simulink subsystem "Lib_QuinIDRxDDC"  (R2023b)
settings: Solver=VariableStepAuto  StartTime=0.0  StopTime=10.0  RelTol=1e-3
values from neighbouring files (symbols this model uses):
  FILT = getFilters(SRC)    [Initialize.m]
undefined symbols (not defined in the file or in its folder): ReaderReceive
libraries: dsphdlfiltering2 x42
settings Model: Creator=NaXin  LastModifiedBy=NaXin

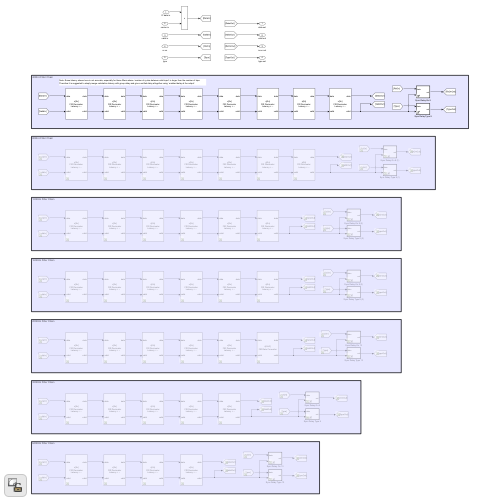
[thumbnail: Simulink's stored preview of the top-level diagram]
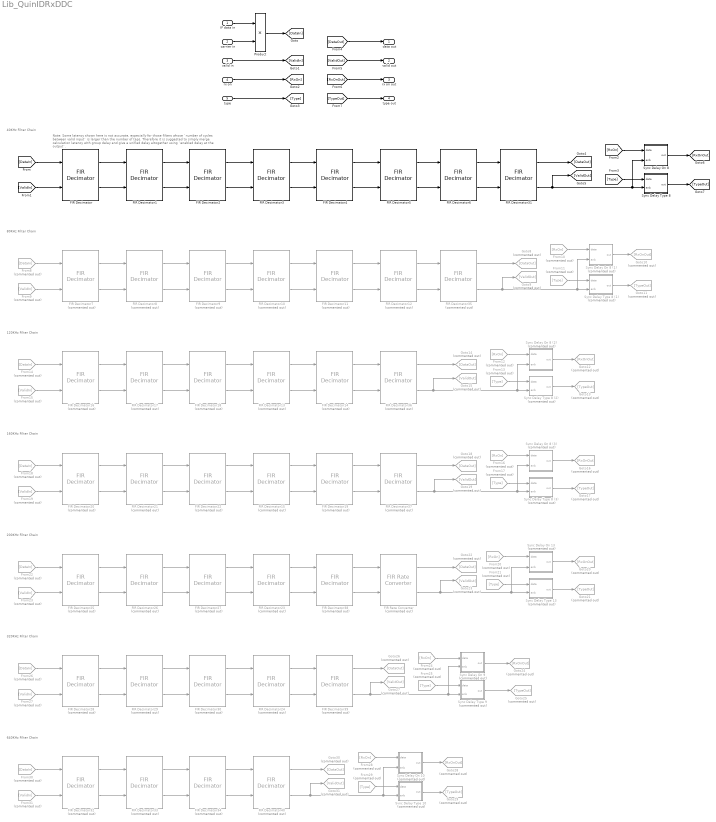
== system Lib_QuinIDRxDDC ==
  note: 40KHz Filter Chain
  note: Note: Some latency shown here is not accurate, especially for those filters whose `number of cycles between valid input` is larger than the number of taps.
      | Therefore it is suggested to simply merge calculation latency with group delay and give a unified delay altogether using `enabled delay at the output`.
  note: 80KHz Filter Chain
  note: 120KHz Filter Chain
  note: 160KHz Filter Chain
  note: 200KHz Filter Chain
  note: 320KHz Filter Chain
  note: 640KHz Filter Chain
  IF data in : Inport
  carrier in : Inport  Port=2
  valid in : Inport  Port=3
  rx on : Inport  Port=4
  type : Inport  Port=5
  FIR Decimator : dsphdlfiltering2/FIR Decimator  Numerator=FILT.Stage1.Numerator  FilterStructure=Direct form systolic  DecimationFactor=FILT.Stage1.DecimationFactor  NumCycles=1  SimulateUsing=Code generation  roundingMode=Round  overflowMode=on  CoefficientsDataTypeStr=fixdt(1,16,15)  OutputDataTypeStr=fixdt(1,16,15)  ResetInputPort=off  HDLGlobalReset=off
  FIR Decimator1 : dsphdlfiltering2/FIR Decimator  Numerator=FILT.Stage2.Numerator  FilterStructure=Direct form systolic  DecimationFactor=FILT.Stage2.DecimationFactor  NumCycles=2  SimulateUsing=Code generation  roundingMode=Round  overflowMode=on  CoefficientsDataTypeStr=fixdt(1,16,15)  OutputDataTypeStr=fixdt(1,16,15)  ResetInputPort=off  HDLGlobalReset=off
  FIR Decimator{10,13,15,23..24,40} (6 alike) : dsphdlfiltering2/FIR Decimator  Commented=on  Numerator=FILT.Stage4.Numerator  FilterStructure=Direct form systolic  DecimationFactor=FILT.Stage4.DecimationFactor  NumCycles=8  SimulateUsing=Code generation  roundingMode=Round  overflowMode=on  CoefficientsDataTypeStr=fixdt(1,16,15)  OutputDataTypeStr=fixdt(1,16,15)  ResetInputPort=off  HDLGlobalReset=off
  FIR Decimator{11,14,19,38..39} (5 alike) : dsphdlfiltering2/FIR Decimator  Commented=on  Numerator=FILT.Stage5.Numerator  FilterStructure=Direct form systolic  DecimationFactor=FILT.Stage5.DecimationFactor  NumCycles=16  SimulateUsing=Code generation  roundingMode=Round  overflowMode=on  CoefficientsDataTypeStr=fixdt(1,16,15)  OutputDataTypeStr=fixdt(1,16,15)  ResetInputPort=off  HDLGlobalReset=off
  FIR Decimator12 : dsphdlfiltering2/FIR Decimator  Commented=on  Numerator=FILT.Stage6.Numerator  FilterStructure=Direct form systolic  DecimationFactor=FILT.Stage6.DecimationFactor  NumCycles=32  SimulateUsing=Code generation  roundingMode=Round  overflowMode=on  CoefficientsDataTypeStr=fixdt(1,16,15)  OutputDataTypeStr=fixdt(1,16,15)  ResetInputPort=off  HDLGlobalReset=off
  FIR Decimator{7,16,20,25,28,32} (6 alike) : dsphdlfiltering2/FIR Decimator  Commented=on  Numerator=FILT.Stage1.Numerator  FilterStructure=Direct form systolic  DecimationFactor=FILT.Stage1.DecimationFactor  NumCycles=1  SimulateUsing=Code generation  roundingMode=Round  overflowMode=on  CoefficientsDataTypeStr=fixdt(1,16,15)  OutputDataTypeStr=fixdt(1,16,15)  ResetInputPort=off  HDLGlobalReset=off
  FIR Decimator{8,17,21,26,29,33} (6 alike) : dsphdlfiltering2/FIR Decimator  Commented=on  Numerator=FILT.Stage2.Numerator  FilterStructure=Direct form systolic  DecimationFactor=FILT.Stage2.DecimationFactor  NumCycles=2  SimulateUsing=Code generation  roundingMode=Round  overflowMode=on  CoefficientsDataTypeStr=fixdt(1,16,15)  OutputDataTypeStr=fixdt(1,16,15)  ResetInputPort=off  HDLGlobalReset=off
  FIR Decimator{9,18,22,27,30,34} (6 alike) : dsphdlfiltering2/FIR Decimator  Commented=on  Numerator=FILT.Stage3.Numerator  FilterStructure=Direct form systolic  DecimationFactor=FILT.Stage3.DecimationFactor  NumCycles=4  SimulateUsing=Code generation  roundingMode=Round  overflowMode=on  CoefficientsDataTypeStr=fixdt(1,16,15)  OutputDataTypeStr=fixdt(1,16,15)  ResetInputPort=off  HDLGlobalReset=off
  FIR Decimator2 : dsphdlfiltering2/FIR Decimator  Numerator=FILT.Stage3.Numerator  FilterStructure=Direct form systolic  DecimationFactor=FILT.Stage3.DecimationFactor  NumCycles=4  SimulateUsing=Code generation  roundingMode=Round  overflowMode=on  CoefficientsDataTypeStr=fixdt(1,16,15)  OutputDataTypeStr=fixdt(1,16,15)  ResetInputPort=off  HDLGlobalReset=off
  FIR Decimator3 : dsphdlfiltering2/FIR Decimator  Numerator=FILT.Stage4.Numerator  FilterStructure=Direct form systolic  DecimationFactor=FILT.Stage4.DecimationFactor  NumCycles=8  SimulateUsing=Code generation  roundingMode=Round  overflowMode=on  CoefficientsDataTypeStr=fixdt(1,16,15)  OutputDataTypeStr=fixdt(1,16,15)  ResetInputPort=off  HDLGlobalReset=off
  FIR Decimator31 : dsphdlfiltering2/FIR Decimator  Numerator=FILT.Stage8.Numerator  FilterStructure=Direct form systolic  DecimationFactor=FILT.Stage8.DecimationFactor  NumCycles=128  SimulateUsing=Code generation  roundingMode=Round  overflowMode=on  CoefficientsDataTypeStr=fixdt(1,16,15)  OutputDataTypeStr=fixdt(1,16,15)  ResetInputPort=off  HDLGlobalReset=off
  FIR Decimator35 : dsphdlfiltering2/FIR Decimator  Commented=on  Numerator=FILT.Stage7.Numerator  FilterStructure=Direct form systolic  DecimationFactor=FILT.Stage7.DecimationFactor  NumCycles=64  SimulateUsing=Code generation  roundingMode=Round  overflowMode=on  CoefficientsDataTypeStr=fixdt(1,16,15)  OutputDataTypeStr=fixdt(1,16,15)  ResetInputPort=off  HDLGlobalReset=off
  FIR Decimator36 : dsphdlfiltering2/FIR Decimator  Commented=on  Numerator=FILT.Stage6.Numerator  FilterStructure=Direct form systolic  DecimationFactor=FILT.Stage6.DecimationFactor  NumCycles=32  SimulateUsing=Code generation  roundingMode=Round  overflowMode=on  CoefficientsDataTypeStr=fixdt(1,16,15)  OutputDataTypeStr=fixdt(1,16,15)  ResetInputPort=off  HDLGlobalReset=off
  FIR Decimator37 : dsphdlfiltering2/FIR Decimator  Commented=on  Numerator=FILT.Stage6.Numerator  FilterStructure=Direct form systolic  DecimationFactor=FILT.Stage6.DecimationFactor  NumCycles=32  SimulateUsing=Code generation  roundingMode=Round  overflowMode=on  CoefficientsDataTypeStr=fixdt(1,16,15)  OutputDataTypeStr=fixdt(1,16,15)  ResetInputPort=off  HDLGlobalReset=off
  FIR Decimator4 : dsphdlfiltering2/FIR Decimator  Numerator=FILT.Stage5.Numerator  FilterStructure=Direct form systolic  DecimationFactor=FILT.Stage5.DecimationFactor  NumCycles=16  SimulateUsing=Code generation  roundingMode=Round  overflowMode=on  CoefficientsDataTypeStr=fixdt(1,16,15)  OutputDataTypeStr=fixdt(1,16,15)  ResetInputPort=off  HDLGlobalReset=off
  FIR Decimator5 : dsphdlfiltering2/FIR Decimator  Numerator=FILT.Stage6.Numerator  FilterStructure=Direct form systolic  DecimationFactor=FILT.Stage6.DecimationFactor  NumCycles=32  SimulateUsing=Code generation  roundingMode=Round  overflowMode=on  CoefficientsDataTypeStr=fixdt(1,16,15)  OutputDataTypeStr=fixdt(1,16,15)  ResetInputPort=off  HDLGlobalReset=off
  FIR Decimator6 : dsphdlfiltering2/FIR Decimator  Numerator=FILT.Stage7.Numerator  FilterStructure=Direct form systolic  DecimationFactor=FILT.Stage7.DecimationFactor  NumCycles=64  SimulateUsing=Code generation  roundingMode=Round  overflowMode=on  CoefficientsDataTypeStr=fixdt(1,16,15)  OutputDataTypeStr=fixdt(1,16,15)  ResetInputPort=off  HDLGlobalReset=off
  FIR Rate Converter : dsphdlfiltering2/FIR Rate Converter  Commented=on  InterpolationFactor=FILT.Stage6.InterpolationFactor  DecimationFactor=FILT.Stage6.DecimationFactor  Numerator=FILT.Stage6.Numerator  SimulateUsing=Code generation  roundingMode=Round  overflowMode=on  CoefficientsDataTypeStr=fixdt(1,16,15)  OutputDataTypeStr=fixdt(1,16,15)  ReadyPort=off
  From{10,12,16,20,24,28} (6 alike) : From  Commented=on  GotoTag=RxOn
  From{11,13,17,21,25,29} (6 alike) : From  Commented=on  GotoTag=Type
  From{8,14,18,22,26,30} (6 alike) : From  Commented=on  GotoTag=DataIn
  From{9,15,19,23,27,31} (6 alike) : From  Commented=on  GotoTag=ValidIn
  Goto{10,12,16,20,24,28} (6 alike) : Goto  Commented=on  GotoTag=RxOnOut
  Goto{11,13,17,21,25,29} (6 alike) : Goto  Commented=on  GotoTag=TypeOut
  Goto{8,14,18,22,26,30} (6 alike) : Goto  Commented=on  GotoTag=DataOut
  Goto{9,15,19,23,27,31} (6 alike) : Goto  Commented=on  GotoTag=ValidOut
  Product : Product  RndMeth=Round  OutDataTypeStr=Inherit: Same as first input
  Sync Delay On 10 : Subsystem  Commented=on
  Sync Delay On 13 : Subsystem  Commented=on
  Sync Delay On 8 : Subsystem
  Sync Delay On 8 (1) : Subsystem  Commented=on
  Sync Delay On 8 (2) : Subsystem  Commented=on
  Sync Delay On 8 (3) : Subsystem  Commented=on
  Sync Delay On 9 : Subsystem  Commented=on
  Sync Delay Type 10 : Subsystem  Commented=on
  Sync Delay Type 13 : Subsystem  Commented=on
  Sync Delay Type 8 : Subsystem
  Sync Delay Type 8 (1) : Subsystem  Commented=on
  Sync Delay Type 8 (2) : Subsystem  Commented=on
  Sync Delay Type 8 (3) : Subsystem  Commented=on
  Sync Delay Type 9 : Subsystem  Commented=on
  data out : Outport
  valid out : Outport  Port=2
  rx on out : Outport  Port=3
  type out : Outport  Port=4
  wires:
  [DataIn] -> FIR Decimator/1
  [ValidIn] -> FIR Decimator/2
  FIR Decimator/2 -> FIR Decimator1/2
  FIR Decimator/1 -> FIR Decimator1/1
  FIR Decimator1/1 -> FIR Decimator2/1
  FIR Decimator1/2 -> FIR Decimator2/2
  FIR Decimator2/1 -> FIR Decimator3/1
  FIR Decimator2/2 -> FIR Decimator3/2
  FIR Decimator3/1 -> FIR Decimator4/1
  FIR Decimator3/2 -> FIR Decimator4/2
  FIR Decimator4/1 -> FIR Decimator5/1
  FIR Decimator4/2 -> FIR Decimator5/2
  FIR Decimator5/1 -> FIR Decimator6/1
  FIR Decimator5/2 -> FIR Decimator6/2
  FIR Decimator6/1 -> FIR Decimator31/1
  FIR Decimator31/2 -> [ValidOut], Sync Delay Type 8/2(enb), Sync Delay On 8/2(enb)
  [RxOn] -> Sync Delay On 8/1(data)
  Sync Delay On 8/1(out) -> [RxOnOut]
  Sync Delay Type 8/1(out) -> [TypeOut]
  [Type] -> Sync Delay Type 8/1(data)
  IF data in/1 -> Product/1
  valid in/1 -> [ValidIn]
  rx on/1 -> [RxOn]
  type/1 -> [Type]
  [DataOut] -> data out/1
  [ValidOut] -> valid out/1
  [RxOnOut] -> rx on out/1
  [TypeOut] -> type out/1
  FIR Decimator9/1 -> FIR Decimator10/1
  Sync Delay On 8 (1)/1(out) -> Goto10/1
  FIR Decimator10/2 -> FIR Decimator11/2
  FIR Decimator9/2 -> FIR Decimator10/2
  From10/1 -> Sync Delay On 8 (1)/1(data)
  FIR Decimator12/1 -> FIR Decimator35/1
  From8/1 -> FIR Decimator7/1
  FIR Decimator11/2 -> FIR Decimator12/2
  FIR Decimator11/1 -> FIR Decimator12/1
  From9/1 -> FIR Decimator7/2
  FIR Decimator8/2 -> FIR Decimator9/2
  FIR Decimator8/1 -> FIR Decimator9/1
  FIR Decimator7/2 -> FIR Decimator8/2
  From11/1 -> Sync Delay Type 8 (1)/1(data)
  FIR Decimator35/2 -> Goto9/1, Sync Delay Type 8 (1)/2(enb), Sync Delay On 8 (1)/2(enb)
  Sync Delay Type 8 (1)/1(out) -> Goto11/1
  FIR Decimator10/1 -> FIR Decimator11/1
  FIR Decimator7/1 -> FIR Decimator8/1
  FIR Decimator36/2 -> Goto15/1, Sync Delay Type 8 (2)/2(enb), Sync Delay On 8 (2)/2(enb)
  FIR Decimator16/1 -> FIR Decimator17/1
  FIR Decimator13/1 -> FIR Decimator14/1
  Sync Delay Type 8 (2)/1(out) -> Goto13/1
  FIR Decimator17/2 -> FIR Decimator18/2
  From13/1 -> Sync Delay Type 8 (2)/1(data)
  FIR Decimator16/2 -> FIR Decimator17/2
  From12/1 -> Sync Delay On 8 (2)/1(data)
  FIR Decimator18/1 -> FIR Decimator13/1
  FIR Decimator18/2 -> FIR Decimator13/2
  From14/1 -> FIR Decimator16/1
  FIR Decimator13/2 -> FIR Decimator14/2
  From15/1 -> FIR Decimator16/2
  Sync Delay On 8 (2)/1(out) -> Goto12/1
  FIR Decimator36/1 -> Goto14/1
  FIR Decimator17/1 -> FIR Decimator18/1
  FIR Decimator22/1 -> FIR Decimator15/1
  From16/1 -> Sync Delay On 8 (3)/1(data)
  FIR Decimator15/2 -> FIR Decimator19/2
  From18/1 -> FIR Decimator20/1
  From17/1 -> Sync Delay Type 8 (3)/1(data)
  FIR Decimator20/2 -> FIR Decimator21/2
  Sync Delay Type 8 (3)/1(out) -> Goto17/1
  FIR Decimator15/1 -> FIR Decimator19/1
  FIR Decimator20/1 -> FIR Decimator21/1
  FIR Decimator37/2 -> Goto19/1, Sync Delay On 8 (3)/2(enb), Sync Delay Type 8 (3)/2(enb)
  FIR Decimator21/1 -> FIR Decimator22/1
  Sync Delay On 8 (3)/1(out) -> Goto16/1
  FIR Decimator22/2 -> FIR Decimator15/2
  From19/1 -> FIR Decimator20/2
  FIR Decimator37/1 -> Goto18/1
  FIR Decimator21/2 -> FIR Decimator22/2
  From23/1 -> FIR Decimator25/2
  FIR Decimator26/2 -> FIR Decimator27/2
  FIR Rate Converter/1 -> Goto22/1
  FIR Decimator27/2 -> FIR Decimator23/2
  FIR Rate Converter/2 -> Goto23/1, Sync Delay On 13/2(enb), Sync Delay Type 13/2(enb)
  FIR Decimator25/2 -> FIR Decimator26/2
  FIR Decimator26/1 -> FIR Decimator27/1
  FIR Decimator38/1 -> FIR Rate Converter/1
  From21/1 -> Sync Delay Type 13/1(data)
  From22/1 -> FIR Decimator25/1
  FIR Decimator25/1 -> FIR Decimator26/1
  Sync Delay On 13/1(out) -> Goto20/1
  From20/1 -> Sync Delay On 13/1(data)
  FIR Decimator38/2 -> FIR Rate Converter/2
  FIR Decimator27/1 -> FIR Decimator23/1
  Sync Delay Type 13/1(out) -> Goto21/1
  Sync Delay Type 9/1(out) -> Goto25/1
  From24/1 -> Sync Delay On 9/1(data)
  FIR Decimator30/1 -> FIR Decimator24/1
  Sync Delay On 9/1(out) -> Goto24/1
  From26/1 -> FIR Decimator28/1
  FIR Decimator28/1 -> FIR Decimator29/1
  From25/1 -> Sync Delay Type 9/1(data)
  FIR Decimator29/1 -> FIR Decimator30/1
  FIR Decimator28/2 -> FIR Decimator29/2
  FIR Decimator29/2 -> FIR Decimator30/2
  From27/1 -> FIR Decimator28/2
  FIR Decimator39/2 -> Goto27/1, Sync Delay On 9/2(enb), Sync Delay Type 9/2(enb)
  FIR Decimator39/1 -> Goto26/1
  FIR Decimator30/2 -> FIR Decimator24/2
  FIR Decimator40/1 -> Goto30/1
  Sync Delay Type 10/1(out) -> Goto29/1
  From29/1 -> Sync Delay Type 10/1(data)
  FIR Decimator32/2 -> FIR Decimator33/2
  From30/1 -> FIR Decimator32/1
  FIR Decimator32/1 -> FIR Decimator33/1
  FIR Decimator33/2 -> FIR Decimator34/2
  From31/1 -> FIR Decimator32/2
  FIR Decimator33/1 -> FIR Decimator34/1
  FIR Decimator40/2 -> Goto31/1, Sync Delay Type 10/2(enb), Sync Delay On 10/2(enb)
  From28/1 -> Sync Delay On 10/1(data)
  Sync Delay On 10/1(out) -> Goto28/1
  FIR Decimator31/1 -> [DataOut]
  FIR Decimator6/2 -> FIR Decimator31/2
  FIR Decimator35/1 -> Goto8/1
  FIR Decimator12/2 -> FIR Decimator35/2
  FIR Decimator14/1 -> FIR Decimator36/1
  FIR Decimator14/2 -> FIR Decimator36/2
  FIR Decimator19/2 -> FIR Decimator37/2
  FIR Decimator19/1 -> FIR Decimator37/1
  FIR Decimator23/2 -> FIR Decimator38/2
  FIR Decimator23/1 -> FIR Decimator38/1
  FIR Decimator24/2 -> FIR Decimator39/2
  FIR Decimator24/1 -> FIR Decimator39/1
  FIR Decimator34/2 -> FIR Decimator40/2
  FIR Decimator34/1 -> FIR Decimator40/1
  carrier in/1 -> Product/2
  Product/1 -> [DataIn]

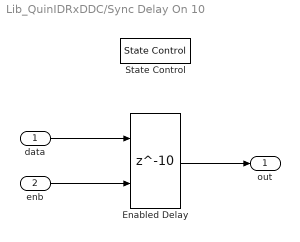
== system Lib_QuinIDRxDDC/Sync Delay On 10 ==
  data : Inport
  enb : Inport  Port=2
  Enabled Delay : Delay  DelayLength=10  InitialCondition=false  ShowEnablePort=on
      settings: InputPortMap=u0,e6
  State Control : StateControl  StateControl=Synchronous
  out : Outport  VectorParamsAs1DForOutWhenUnconnected=off
  wires:
  data/1 -> Enabled Delay/1
  Enabled Delay/1 -> out/1
  enb/1 -> Enabled Delay/2

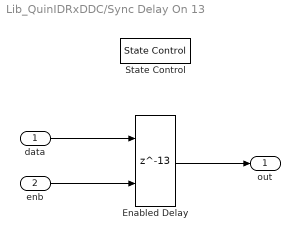
== system Lib_QuinIDRxDDC/Sync Delay On 13 ==
  data : Inport
  enb : Inport  Port=2
  Enabled Delay : Delay  DelayLength=13  InitialCondition=false  ShowEnablePort=on
      settings: InputPortMap=u0,e6
  State Control : StateControl  StateControl=Synchronous
  out : Outport  VectorParamsAs1DForOutWhenUnconnected=off
  wires:
  data/1 -> Enabled Delay/1
  Enabled Delay/1 -> out/1
  enb/1 -> Enabled Delay/2

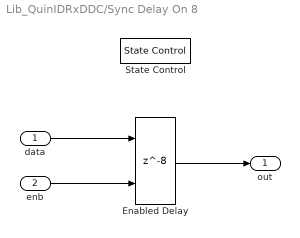
== system Lib_QuinIDRxDDC/Sync Delay On 8 ==
  data : Inport
  enb : Inport  Port=2
  Enabled Delay : Delay  DelayLength=8  InitialCondition=false  ShowEnablePort=on
      settings: InputPortMap=u0,e6
  State Control : StateControl  StateControl=Synchronous
  out : Outport  VectorParamsAs1DForOutWhenUnconnected=off
  wires:
  data/1 -> Enabled Delay/1
  Enabled Delay/1 -> out/1
  enb/1 -> Enabled Delay/2

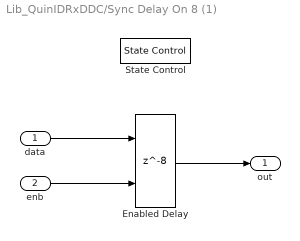
== system Lib_QuinIDRxDDC/Sync Delay On 8 (1) ==
  data : Inport
  enb : Inport  Port=2
  Enabled Delay : Delay  DelayLength=8  InitialCondition=false  ShowEnablePort=on
      settings: InputPortMap=u0,e6
  State Control : StateControl  StateControl=Synchronous
  out : Outport  VectorParamsAs1DForOutWhenUnconnected=off
  wires:
  Enabled Delay/1 -> out/1
  data/1 -> Enabled Delay/1
  enb/1 -> Enabled Delay/2

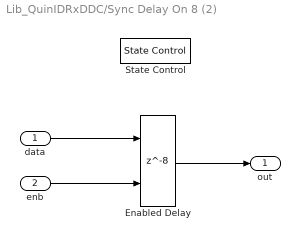
== system Lib_QuinIDRxDDC/Sync Delay On 8 (2) ==
  data : Inport
  enb : Inport  Port=2
  Enabled Delay : Delay  DelayLength=8  InitialCondition=false  ShowEnablePort=on
      settings: InputPortMap=u0,e6
  State Control : StateControl  StateControl=Synchronous
  out : Outport  VectorParamsAs1DForOutWhenUnconnected=off
  wires:
  Enabled Delay/1 -> out/1
  data/1 -> Enabled Delay/1
  enb/1 -> Enabled Delay/2

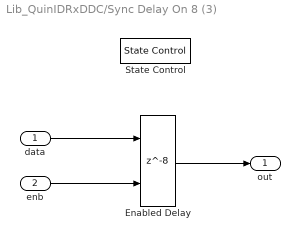
== system Lib_QuinIDRxDDC/Sync Delay On 8 (3) ==
  data : Inport
  enb : Inport  Port=2
  Enabled Delay : Delay  DelayLength=8  InitialCondition=false  ShowEnablePort=on
      settings: InputPortMap=u0,e6
  State Control : StateControl  StateControl=Synchronous
  out : Outport  VectorParamsAs1DForOutWhenUnconnected=off
  wires:
  data/1 -> Enabled Delay/1
  Enabled Delay/1 -> out/1
  enb/1 -> Enabled Delay/2

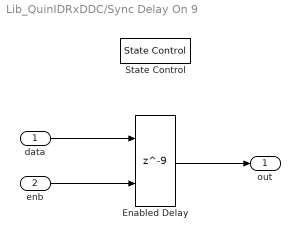
== system Lib_QuinIDRxDDC/Sync Delay On 9 ==
  data : Inport
  enb : Inport  Port=2
  Enabled Delay : Delay  DelayLength=9  InitialCondition=false  ShowEnablePort=on
      settings: InputPortMap=u0,e6
  State Control : StateControl  StateControl=Synchronous
  out : Outport  VectorParamsAs1DForOutWhenUnconnected=off
  wires:
  data/1 -> Enabled Delay/1
  Enabled Delay/1 -> out/1
  enb/1 -> Enabled Delay/2

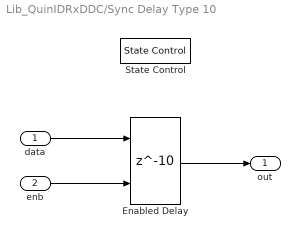
== system Lib_QuinIDRxDDC/Sync Delay Type 10 ==
  data : Inport
  enb : Inport  Port=2
  Enabled Delay : Delay  DelayLength=10  InitialCondition=ReaderReceive.RN16  ShowEnablePort=on
      settings: InputPortMap=u0,e6
  State Control : StateControl  StateControl=Synchronous
  out : Outport  VectorParamsAs1DForOutWhenUnconnected=off
  wires:
  data/1 -> Enabled Delay/1
  Enabled Delay/1 -> out/1
  enb/1 -> Enabled Delay/2

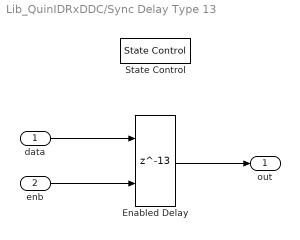
== system Lib_QuinIDRxDDC/Sync Delay Type 13 ==
  data : Inport
  enb : Inport  Port=2
  Enabled Delay : Delay  DelayLength=13  InitialCondition=ReaderReceive.RN16  ShowEnablePort=on
      settings: InputPortMap=u0,e6
  State Control : StateControl  StateControl=Synchronous
  out : Outport  VectorParamsAs1DForOutWhenUnconnected=off
  wires:
  data/1 -> Enabled Delay/1
  Enabled Delay/1 -> out/1
  enb/1 -> Enabled Delay/2

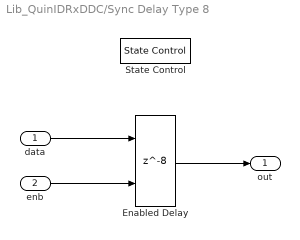
== system Lib_QuinIDRxDDC/Sync Delay Type 8 ==
  data : Inport
  enb : Inport  Port=2
  Enabled Delay : Delay  DelayLength=8  InitialCondition=ReaderReceive.RN16  ShowEnablePort=on
      settings: InputPortMap=u0,e6
  State Control : StateControl  StateControl=Synchronous
  out : Outport  VectorParamsAs1DForOutWhenUnconnected=off
  wires:
  data/1 -> Enabled Delay/1
  Enabled Delay/1 -> out/1
  enb/1 -> Enabled Delay/2

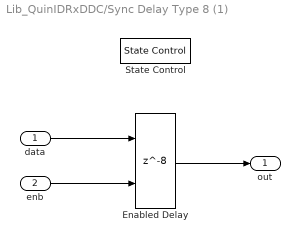
== system Lib_QuinIDRxDDC/Sync Delay Type 8 (1) ==
  data : Inport
  enb : Inport  Port=2
  Enabled Delay : Delay  DelayLength=8  InitialCondition=ReaderReceive.RN16  ShowEnablePort=on
      settings: InputPortMap=u0,e6
  State Control : StateControl  StateControl=Synchronous
  out : Outport  VectorParamsAs1DForOutWhenUnconnected=off
  wires:
  data/1 -> Enabled Delay/1
  Enabled Delay/1 -> out/1
  enb/1 -> Enabled Delay/2

== system Lib_QuinIDRxDDC/Sync Delay Type 8 (2) ==
  data : Inport
  enb : Inport  Port=2
  Enabled Delay : Delay  DelayLength=8  InitialCondition=ReaderReceive.RN16  ShowEnablePort=on
      settings: InputPortMap=u0,e6
  State Control : StateControl  StateControl=Synchronous
  out : Outport  VectorParamsAs1DForOutWhenUnconnected=off
  wires:
  data/1 -> Enabled Delay/1
  Enabled Delay/1 -> out/1
  enb/1 -> Enabled Delay/2

== system Lib_QuinIDRxDDC/Sync Delay Type 8 (3) ==
  data : Inport
  enb : Inport  Port=2
  Enabled Delay : Delay  DelayLength=8  InitialCondition=ReaderReceive.RN16  ShowEnablePort=on
      settings: InputPortMap=u0,e6
  State Control : StateControl  StateControl=Synchronous
  out : Outport  VectorParamsAs1DForOutWhenUnconnected=off
  wires:
  data/1 -> Enabled Delay/1
  Enabled Delay/1 -> out/1
  enb/1 -> Enabled Delay/2

== system Lib_QuinIDRxDDC/Sync Delay Type 9 ==
  data : Inport
  enb : Inport  Port=2
  Enabled Delay : Delay  DelayLength=9  InitialCondition=ReaderReceive.RN16  ShowEnablePort=on
      settings: InputPortMap=u0,e6
  State Control : StateControl  StateControl=Synchronous
  out : Outport  VectorParamsAs1DForOutWhenUnconnected=off
  wires:
  data/1 -> Enabled Delay/1
  Enabled Delay/1 -> out/1
  enb/1 -> Enabled Delay/2
